simulink model "cep_SIM"  (R2022b)
settings: Solver=VariableStepAuto  StartTime=0.0  StopTime=10.0  RelTol=1e-3
values from neighbouring files (symbols this model uses):
  A = [-1.064 1.000; 290.26 0.00]    [cep.m]
  B = [-0.25; -331.40]    [cep.m]
  C = [-123.34 0.00; 0.00 1.00]    [cep.m]
  D = [-13.51; 0]    [cep.m]
  dT1 = 0.75    [cep.m]
  dT2 = 0.25    [cep.m]
  ELEV_INIT = 10000    [cep.m]
  ELEV_TARGET = 795    [cep.m]
  LAT_INIT = 34.2329    [cep.m]
  LAT_OBS = 34.61916    [cep.m]
  LAT_TARGET = 34.6588    [cep.m]
  LON_INIT = -119.4573    [cep.m]
  LON_OBS = -118.8429    [cep.m]
  LON_TARGET = -118.769745    [cep.m]
  Vel = 1021.08    [cep.m]
undefined symbols (not defined in the file or in its folder): Earth, K, L, WGS84
libraries: simulink x3, slpidlib x1, aerolibtransform2 x1, aerolibanimutils x1
settings Model: Creator=Fame Computers  LastModifiedBy=Dusk Treader

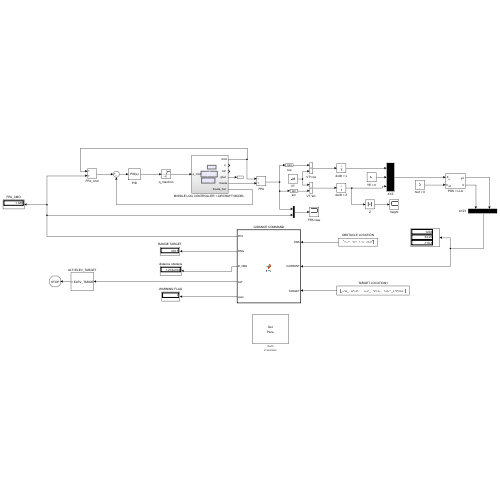
[thumbnail: Simulink's stored preview of the top-level diagram]
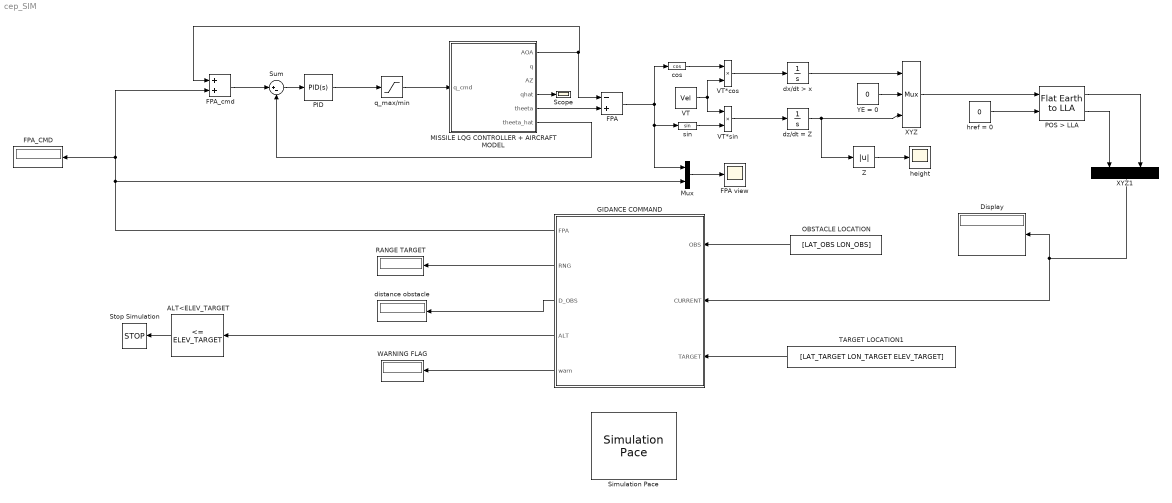
== system cep_SIM ==
  ALT<ELEV_TARGET : simulink/Logic and Bit Operations/Compare To Constant  relop=<=  const=ELEV_TARGET  OutDataTypeStr=boolean
  Display : Display
  FPA : Sum  Inputs=-+
  FPA view : Scope
  FPA_CMD : Display
  FPA_cmd : Sum
  GIDANCE COMMAND : MATLAB Function  TreatAsAtomicUnit=on
  "MISSILE LQG CONTROLLER + AIRCRAFT MODEL  " : Subsystem
  Mux : Mux  Inputs=2
  OBSTACLE LOCATION : Constant  Value=[LAT_OBS LON_OBS]
  PID : slpidlib/PID Controller  Controller=PID  Form=Parallel  TimeDomain=Continuous-time  UseExternalTs=off  SampleTime=-1  IntegratorMethod=Forward Euler  FilterMethod=Forward Euler  ControllerParametersSource=internal  P=-1  I=0  UseKiTs=off  D=0  N=100  UseFilter=on  TunerSelectOption=Transfer Function Based (PID Tuner App)  InitialConditionSource=internal  InitialConditionForIntegrator=0  InitialConditionForFilter=0  DifferentiatorICPrevScaledInput=0  ExternalReset=none  TrackingMode=off  Kt=1  LimitOutput=off  SatLimitsSource=internal  UpperSaturationLimit=inf  LowerSaturationLimit=-inf  LinearizeAsGain=on  AntiWindupMode=none  Kb=1  LimitIntegrator=off  UpperIntegratorSaturationLimit=inf  LowerIntegratorSaturationLimit=-inf  POutMin=[]  POutMax=[]  IOutMin=[]  IOutMax=[]  DOutMin=[]  DOutMax=[]  NOutMin=[]  NOutMax=[]  SumOutMin=[]  SumOutMax=[]  SaturationOutMin=[]  SaturationOutMax=[]  PParamMin=[]  PParamMax=[]  IParamMin=[]  IParamMax=[]  DParamMin=[]  DParamMax=[]  NParamMin=[]  NParamMax=[]  KbParamMin=[]  KbParamMax=[]  KtParamMin=[]  KtParamMax=[]  KbOutMin=[]  KbOutMax=[]  KtOutMin=[]  KtOutMax=[]  IntegratorOutMin=[]  IntegratorOutMax=[]  FilterOutMin=[]  FilterOutMax=[]  SumI1OutMin=[]  SumI1OutMax=[]  SumI2OutMin=[]  SumI2OutMax=[]  SumI3OutMin=[]  SumI3OutMax=[]  SumI4OutMin=[]  SumI4OutMax=[]  SumDOutMin=[]  SumDOutMax=[]  DifferentiatorOutMin=[]  DifferentiatorOutMax=[]  FilterDiffOutCoefMin=[]  FilterDiffOutCoefMax=[]  ReciprocalOutMin=[]  ReciprocalOutMax=[]  SumDenOutMin=[]  SumDenOutMax=[]  SumNumOutMin=[]  SumNumOutMax=[]  DivideOutMin=[]  DivideOutMax=[]  UdiffTsProdOutMin=[]  UdiffTsProdOutMax=[]  NTsProdOutMin=[]  NTsProdOutMax=[]  UintegralTsProdOutMin=[]  UintegralTsProdOutMax=[]  UngainTsProdOutMin=[]  UngainTsProdOutMax=[]  ClampingZeroOutDataTypeStr=Inherit: Inherit via back propagation  ClampingZeroOutMin=[]  ClampingZeroOutMax=[]  FilterDenConstantOutDataTypeStr=Inherit: Inherit via back propagation  FilterDenConstantOutMin=[]  FilterDenConstantOutMax=[]  PCopyOutDataTypeStr=Inherit: Inherit via back propagation  PCopyOutMin=[]  PCopyOutMax=[]  NCopyOutDataTypeStr=Inherit: Inherit via back propagation  NCopyOutMin=[]  NCopyOutMax=[]  IntegratorContinuousStateAttributes=''  IntegratorStateMustResolveToSignalObject=off  IntegratorRTWStateStorageClass=Auto  FilterContinuousStateAttributes=''  FilterStateMustResolveToSignalObject=off  FilterRTWStateStorageClass=Auto  ParallelPVariant=InternalParameters  IdealPVariant=Disabled  IVariant=InternalParameters  DVariant=InternalParameters  IntegratorVariant=Continuous  SatVariant=Disabled  AWVariant=Passthrough  PCopyVariant=Disabled  TRVariant=Disabled  FdbkBlocksVariant=Forward  IdealPFdbkVariant=Disabled  SatFdbkVariant=Disabled  DerivativeFilterVariant=ContFilter  NVariant=InternalParameters  NCopyVariant=Disabled  FilterICVariant=InternalICsFilter  IntegratorICVariant=InternalICs  ExternalResetVariant=Disabled  TRSumVariant=Passthrough  SumFdbkVariant=Disabled  SumVariant=Sum_PID  TsampFilterVariant=InternalTs  TsampNgainVariant=Passthrough  TsampIntegralVariant=Passthrough  ExternalSaturationOutDataTypeStr=Inherit: Same as second input
  POS > LLA : aerolibtransform2/Flat Earth to LLA  units=Metric (MKS)  ptype=Earth (WGS84)  F=1/298.257223563  R=6378137  refPosPort=off  LL0=[LAT_INIT LON_INIT]  psi=yaw_init
  RANGE TARGET : Display
  Scope : Scope
  Simulation Pace : aerolibanimutils/Simulation Pace  SimulationPace=2  SleepMode=Auto  OutputPaceError=off  SampleTime=1/30
  Stop Simulation : Stop
  Sum : Sum  Inputs=|+-
  TARGET LOCATION1 : Constant  Value=[LAT_TARGET LON_TARGET ELEV_TARGET]
  VT : Constant  Value=Vel
  VT*cos : Product
  VT*sin : Product
  WARNING FLAG : Display
  XYZ : Mux  Inputs=3
  XYZ1 : Mux  Inputs=2
  YE = 0 : Constant  Value=0
  Z : Abs  SaturateOnIntegerOverflow=off
  cos : Trigonometry  Operator=cos
  distance obstacle : Display
  dx/dt > x : Integrator
  dz/dt = Z : Integrator  InitialCondition=-ELEV_INIT
  height : Scope
  href = 0 : Constant  Value=0
  q_max/min : Saturate
  sin : Trigonometry
  wires:
  PID/1 -> q_max/min/1
  q_max/min/1 -> "MISSILE LQG CONTROLLER + AIRCRAFT MODEL  "/1(q_cmd)
  Sum/1 -> PID/1
  "MISSILE LQG CONTROLLER + AIRCRAFT MODEL  "/6("theeta_hat  ") -> Sum/2
  FPA_cmd/1 -> Sum/1
  "MISSILE LQG CONTROLLER + AIRCRAFT MODEL  "/1(AOA) -> FPA/1, FPA_cmd/1
  "MISSILE LQG CONTROLLER + AIRCRAFT MODEL  "/5(theeta) -> FPA/2
  GIDANCE COMMAND/1(FPA) -> Mux/2, FPA_CMD/1, FPA_cmd/2
  Mux/1 -> FPA view/1
  FPA/1 -> cos/1, sin/1, Mux/1
  sin/1 -> VT*sin/2
  cos/1 -> VT*cos/1
  VT/1 -> VT*sin/1, VT*cos/2
  VT*cos/1 -> dx/dt > x/1
  VT*sin/1 -> dz/dt = Z/1
  dz/dt = Z/1 -> Z/1, XYZ/3
  dx/dt > x/1 -> XYZ/1
  YE = 0/1 -> XYZ/2
  Z/1 -> height/1
  XYZ/1 -> POS > LLA/1
  href = 0/1 -> POS > LLA/2
  POS > LLA/2 -> XYZ1/1
  POS > LLA/1 -> XYZ1/2
  OBSTACLE LOCATION/1 -> GIDANCE COMMAND/1(OBS)
  TARGET LOCATION1/1 -> GIDANCE COMMAND/3(TARGET)
  XYZ1/1 -> Display/1, GIDANCE COMMAND/2(CURRENT)
  GIDANCE COMMAND/2(RNG) -> RANGE TARGET/1
  GIDANCE COMMAND/3(D_OBS) -> distance obstacle/1
  GIDANCE COMMAND/5(warn) -> WARNING FLAG/1
  GIDANCE COMMAND/4(ALT) -> ALT<ELEV_TARGET/1
  ALT<ELEV_TARGET/1 -> Stop Simulation/1
  "MISSILE LQG CONTROLLER + AIRCRAFT MODEL  "/4("qhat  ") -> Scope/1

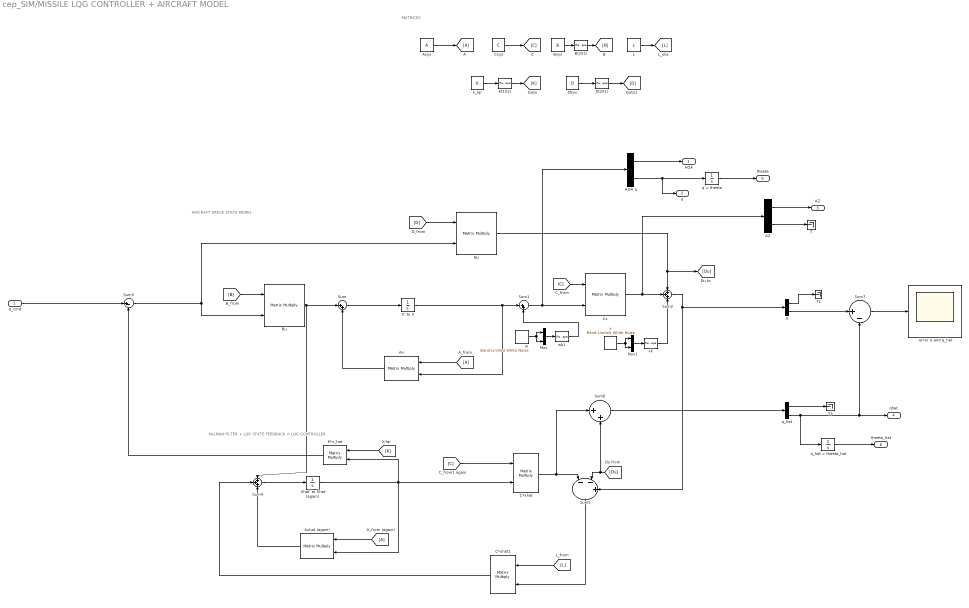
== system cep_SIM/MISSILE LQG CONTROLLER + AIRCRAFT MODEL   ==
  note: KALMAN FILTER + LQR STATE FEEDBACK = LQG CONTROLLER
  note: AIRCRAFT SPACE STATE MODEL
  note: MATRICES
  q_cmd : Inport
  A : Goto
  AOA q : Demux  Outputs=2
  AZ : Demux  Outputs=2
  A_from : From
  A_from (again) : From
  Asys : Constant  Value=A
  Ax : Product  Multiplication=Matrix(*)
  Axhat (again) : Product  Multiplication=Matrix(*)
  B(2X1) : Reshape  OutputDimensionality=Customize  OutputDimensions=[2,1]
  Bsys : Constant  Value=B
  Bu : Product  Multiplication=Matrix(*)
  C*xhat : Product  Multiplication=Matrix(*)
  C*xhat1 : Product  Multiplication=Matrix(*)
  Csys : Constant  Value=C
  Cx : Product  Multiplication=Matrix(*)
  "D(2X1) " : Reshape  OutputDimensionality=Customize  OutputDimensions=[2,1]
  Dsys : Constant  Value=D
  Du : Product  Multiplication=Matrix(*)
  K(1X2) : Reshape  OutputDimensionality=Customize  OutputDimensions=[1,2]
  K*x_hat : Product  Multiplication=Matrix(*)
  L : Constant  Value=L
  Mux : Mux  Inputs=2
  Mux1 : Mux  Inputs=2
  Sum : Sum  Inputs=|++
  Sum1 : Sum  Inputs=|++
  Sum2 : Sum  Inputs=+++
  Sum3 : Sum  Inputs=|+-
  Sum4 : Sum  Inputs=+++
  Sum5 : Sum  Inputs=|--+
  Sum6 : Sum  Inputs=|++
  Sum7 : Sum  Inputs=|+-
  T : Terminator
  T1 : Terminator
  T3 : Terminator
  X' to X : Integrator
  Xhat' to Xhat (again) : Integrator
  error q and q_hat : Scope
  k_lqr : Constant  Value=K
  q : Demux  Outputs=2
  q > theeta : Integrator
  q_hat : Demux  Outputs=2
  q_hat > theeta_hat : Integrator
  v : simulink/Sources/Band-Limited White Noise  Cov=[0.00001]  Ts=dT2  seed=[23341]
  vk : Reshape  OutputDimensionality=Customize  OutputDimensions=[2,1]
  w : simulink/Sources/Band-Limited White Noise  Cov=[0.00000001]  Ts=dT1  seed=[23341]
  wk1 : Reshape  OutputDimensionality=Customize  OutputDimensions=[2,1]
  AOA : Outport
  "q  " : Outport  Port=2
  "AZ  " : Outport  Port=3
  "qhat  " : Outport  Port=4
  theeta : Outport  Port=5
  "theeta_hat  " : Outport  Port=6
  wires:
  A_from/1 -> Ax/1
  Sum2/1 -> q/1, Sum5/3
  q_hat > theeta_hat/1 -> "theeta_hat  "/1
  [D] -> Du/1
  "D(2X1) "/1 -> [D]
  w/1 -> Mux/2, Mux/1
  wk1/1 -> Sum1/2
  C*xhat/1 -> Sum6/1, Sum5/1
  vk/1 -> Sum2/3
  [Du] -> Sum5/2, Sum6/2
  Axhat (again)/1 -> Sum4/3
  Du/1 -> [Du], Sum2/1
  q_cmd/1 -> Sum3/1
  Dsys/1 -> "D(2X1) "/1
  Sum5/1 -> C*xhat1/2
  Bu/1 -> Sum/1, Sum4/1
  K*x_hat/1 -> Sum3/2
  q/1 -> T1/1
  C*xhat1/1 -> Sum4/2
  q_hat/1 -> T3/1
  q > theeta/1 -> theeta/1
  Sum7/1 -> error q and q_hat/1
  v/1 -> Mux1/2, Mux1/1
  AOA q/1 -> AOA/1
  Xhat' to Xhat (again)/1 -> K*x_hat/2, Axhat (again)/2, C*xhat/2
  X' to X/1 -> Ax/2, Sum1/1
  Sum/1 -> X' to X/1
  AZ/1 -> "AZ  "/1
  q_hat/2 -> q_hat > theeta_hat/1, "qhat  "/1, Sum7/2
  AOA q/2 -> "q  "/1, q > theeta/1
  Sum1/1 -> Cx/2, AOA q/1
  B(2X1)/1 -> [B]
  K(1X2)/1 -> [K]
  [K] -> K*x_hat/1
  Sum3/1 -> Bu/2, Du/2
  Sum6/1 -> q_hat/1
  AZ/2 -> T/1
  Mux1/1 -> vk/1
  [L] -> C*xhat1/1
  q/2 -> Sum7/1
  Cx/1 -> AZ/1, Sum2/2
  Mux/1 -> wk1/1
  k_lqr/1 -> K(1X2)/1
  [C] -> C*xhat/1
  [B] -> Bu/1
  Sum4/1 -> Xhat' to Xhat (again)/1
  L/1 -> [L]
  Ax/1 -> Sum/2
  Bsys/1 -> B(2X1)/1
  A_from (again)/1 -> Axhat (again)/1
  Asys/1 -> A/1
  Csys/1 -> [C]
  [C] -> Cx/1

== matlab function cep_SIM/GIDANCE COMMAND ==
  data: OBS input; FPA output; CURRENT input; TARGET input; RNG output; D_OBS output; ALT output; warn output
function [FPA,RNG,D_OBS,ALT,warn] = fcn(OBS, CURRENT, TARGET)


R = 6.371e3; 
d2r = pi/180;
%OBSTACLE LOCATION
LAT_OBS=OBS(1);
LON_OBS=OBS(2);
%OBSTACLE THRESHOLD (ZONE)
thres=2000;
%TARGET LOCATION
LAT_TARGET=TARGET(1);
LON_TARGET=TARGET(2);
ELEV_TARGET=TARGET(3)
%CURRENT LOCATION
ELEV_CUR=CURRENT(1);
LAT_CUR=CURRENT(2);
LON_CUR=CURRENT(3);
% % distance to target
l1= LAT_CUR*d2r;
u1 =LON_CUR*d2r;
l2 =LAT_TARGET*d2r;
u2 =LON_TARGET*d2r;
dh = abs(ELEV_TARGET-ELEV_CUR);

dl =l2-l1;
du =u2-u1;

a = sin(dl/2)^2 + cos(l1)*cos(l2)*sin(du/2)^2;
c = 2*atan2(sqrt(a),sqrt(1-a));
d = R*c; %horizontal distance (in m)

% % distance from obstacle
l3= LAT_OBS*d2r;
u3 = LON_OBS*d2r;
dl = l3-l1;
du=u3-u1;
a = sin(dl/2)^2 + cos(l1)*cos(l2)*sin(du/2)^2;
c = 2*atan2(sqrt(a), sqrt(1-a));
d_obs = R*c; %horizontal distance (in m)

% %  current range (from target)  range> distance
range=sqrt(d^2+dh^2);
% % calculate command flight path set point based on d.obs range
if abs(d_obs)>=thres
    w=0;
    FPA_CMD=atan(dh/d);
else
     w=1;
    FPA_CMD=0;
end

% % output variables
FPA = FPA_CMD;
RNG = range;
D_OBS = d_obs;
warn = w;
ALT = ELEV_CUR;
